simulink model "Simulation_NoVI"  (R2022b)
settings: Solver=VariableStepAuto  StartTime=0.0  StopTime=25  RelTol=1e-3
values from neighbouring files (symbols this model uses):
  A = [0 1 1 1 ; 1 0 1 1 ; 1 1 0 1 ; 1 1 1 0]    [Primary_test1.m]    (also in init.mat = [0 1 1 1 1 0 1 1 1 1 0 1 ... (16 elements, 4x4)])
  C_f = 0.000112315*9    (= 0.001010835)    [Main.m]    (also in PSO_2paras.m = swarm(i,2); PSO_filter_2paras.m = swarm(i,2)/10000; Primary_test1.m; Script_18June.m = 0.0112315)
  f_c = 50e3    (= 50000)    [Main.m]    (also in Primary_test1.m; Script_18June.m; Script_23June.m; Script_5thJune.m)
  k = -0.5    [Main.m]    (also in Primary_test1.m; Savedata.m = 0.2909; Script_18June.m = 0.5; Script_23June.m)
  K_h11 = 0    [Main.m]    (also in PSO_HC.m = swarm(i,4); Primary_test1.m; Script_18June.m; Script_23June.m)
  K_h13 = 0    [Main.m]    (also in Primary_test1.m; Script_18June.m; Script_23June.m; Script_5thJune.m)
  K_h5 = 0    [Main.m]    (also in PSO_HC.m = swarm(i,1); Primary_test1.m = 1; Script_18June.m; Script_23June.m)
  K_h7 = 0    [Main.m]    (also in PSO_HC.m = swarm(i,2); Primary_test1.m; Script_18June.m; Script_23June.m)
  K_h9 = 0    [Main.m]    (also in PSO_HC.m = swarm(i,3); Script_18June.m; Script_23June.m; Script_5thJune.m)
  ki_pr = 160    [Main.m]    (also in PSO.m = swarm(i,2); Primary_test1.m; Savedata.m = 422.4716; Script_18June.m = 150)
  kL = 1e-7    (= 1e-07)    [Main.m]    (also in Primary_test1.m; Script_18June.m; Script_23June.m; Script_5thJune.m)
  Kp_pr = 1.7    [Main.m]    (also in PSO.m = swarm(i,1); Primary_test1.m; Savedata.m = 0.9028; Script_18June.m = 1)
  L_f = 0.000659829*1.4    (= 0.0009237606)    [Main.m]    (also in PSO_2paras.m = swarm(i,1); PSO_filter_2paras.m = swarm(i,1); Primary_test1.m; Script_18June.m = 0.000295603392)
  L_in1 = 0.35e-3    (= 0.00035)    [Main.m]    (also in Primary_test1.m; Script_18June.m; Script_23June.m; Script_5thJune.m)
  L_in2 = 0.35e-3    (= 0.00035)    [Main.m]    (also in Primary_test1.m; Script_18June.m; Script_23June.m; Script_5thJune.m)
  L_in3 = 0.35e-3    (= 0.00035)    [Main.m]    (also in Primary_test1.m; Script_18June.m; Script_23June.m; Script_5thJune.m)
  L_in4 = 0.35e-3    (= 0.00035)    [Main.m]    (also in Primary_test1.m; Script_18June.m; Script_23June.m; Script_5thJune.m)
  lambda1 = 5.5*[1 1 0.8 0.8]'    [Primary_test1.m]    (also in init.mat = [5.5 5.5 4.4 4.4])
  lambda2 = 30.5*[0.8e-2 0.8e-2 0.5e-2 0.5e-2]'    [Primary_test1.m]    (also in init.mat = [0.244 0.244 0.1525 0.1525])
  lambda3 = 62.5*[1.5e-3 1.5e-3 1e-3 1.1e-3]'    [Primary_test1.m]    (also in init.mat = [0.09375 0.09375 0.0625 0.06875])
  LD_ref1 = 100e-6    (= 0.0001)    [Main.m]    (also in Primary_test1.m; Script_18June.m = 5e-05; Script_23June.m = 1e-05; Script_5thJune.m = 1e-05)
  lo_co = 0.1    [Main.m]    (also in Primary_test1.m; Script_18June.m; Script_23June.m; Script_5thJune.m)
  load_off = 10    [Main.m]    (also in Primary_test1.m = 2; Script_18June.m = 28; Script_23June.m = 28; Script_5thJune.m)
  load_on = 0.21    [Main.m]    (also in Primary_test1.m = 1; Script_18June.m; Script_23June.m; Script_5thJune.m)
  m_p1 = 9.4e-5/droopDivide    (= 9.4e-06)    [Main.m]    (also in Primary_test1.m; Script_18June.m = 9.4e-05; Script_23June.m = 9.4e-05; Script_5thJune.m = 5e-05)
  m_p2 = 9.4e-5/droopDivide    (= 9.4e-06)    [Main.m]    (also in Primary_test1.m; Script_18June.m = 9.4e-05; Script_23June.m = 9.4e-05; Script_5thJune.m = 5e-05)
  m_p3 = 11.4e-5/droopDivide    (= 1.14e-05)    [Main.m]    (also in Primary_test1.m; Script_18June.m = 0.000114; Script_23June.m = 0.000114; Script_5thJune.m = 6.42857142857e-05)
  m_p4 = 11.4e-5/droopDivide    (= 1.14e-05)    [Main.m]    (also in Primary_test1.m; Script_18June.m = 0.000114; Script_23June.m = 0.000114; Script_5thJune.m = 6.42857142857e-05)
  N = 2    [Primary_test1.m]    (also in init.mat)
  n_q1 = 1.3e-3/droopDivide2    (= 6.5e-05)    [Main.m]    (also in Primary_test1.m; Script_18June.m; Script_23June.m; Script_5thJune.m = 0.2)
  n_q2 = 1.3e-3/droopDivide2    (= 6.5e-05)    [Main.m]    (also in Primary_test1.m; Script_18June.m; Script_23June.m; Script_5thJune.m = 0.2)
  n_q3 = 1.5e-3/droopDivide2    (= 7.5e-05)    [Main.m]    (also in Primary_test1.m; Script_18June.m; Script_23June.m; Script_5thJune.m = 0.257142857143)
  n_q4 = 1.5e-3/droopDivide2    (= 7.5e-05)    [Main.m]    (also in Primary_test1.m; Script_18June.m; Script_23June.m; Script_5thJune.m = 0.257142857143)
  Pmax = [45e3 45e3 37e3 37e3]'    [Primary_test1.m]    (also in init.mat = [45000 45000 37000 37000])
  PMW = V_nom/0.55    [Main.m]    (also in Primary_test1.m; Script_18June.m = V_nom/0.4; Script_23June.m; Script_5thJune.m = 220*sqrt(2))
  R_f = 0.35    [Main.m]    (also in PSO_filter_2paras.m = 10*L_f; Primary_test1.m; Savedata.m = 0.249593207053; Script_18June.m = 0.1)
  R_in1 = 0.03    [Main.m]    (also in Primary_test1.m; Script_18June.m; Script_23June.m; Script_5thJune.m)
  R_in2 = 0.03    [Main.m]    (also in Primary_test1.m; Script_18June.m; Script_23June.m; Script_5thJune.m)
  R_in3 = 0.03    [Main.m]    (also in Primary_test1.m; Script_18June.m; Script_23June.m; Script_5thJune.m)
  R_in4 = 0.03    [Main.m]    (also in Primary_test1.m; Script_18June.m; Script_23June.m; Script_5thJune.m)
  time_thresh = 0.2    [Main.m]    (also in Primary_test1.m; Script_18June.m; Script_23June.m; Script_5thJune.m)
  Ts = 10e-6    (= 1e-05)    [Main.m]    (also in Primary_test1.m; Script_18June.m; Script_23June.m; Script_5thJune.m)
  Tsamp = 0.1    [Primary_test1.m]    (also in init.mat)
  V_nom = 220*sqrt(2)    [Main.m]    (also in Primary_test1.m; Script_18June.m; Script_23June.m; Script_5thJune.m)
  Vdc = 600    [Main.m]    (also in Primary_test1.m; Script_18June.m; Script_23June.m; Script_5thJune.m)
  w_c_high = 2*pi*50    (= 314.159265359)    [Main.m]    (also in Primary_test1.m; Script_18June.m = 307.876080052; Script_23June.m; Script_5thJune.m = 307.876080052)
  w_nom = 2*pi*f    (= 314.159265359)    [Main.m]    (also in Primary_test1.m; Script_18June.m; Script_23June.m; Script_5thJune.m)
  wc_hc = 1    [Main.m]    (also in Primary_test1.m; Script_18June.m = 0.3; Script_23June.m; Script_5thJune.m = 0.3)
  wc_pr = 3    [Main.m]    (also in PSO.m = swarm(i,3); Primary_test1.m; Savedata.m = 1.36672; Script_18June.m = 1.5)
undefined symbols (not defined in the file or in its folder): DiscIntNeverNeededParam, i
libraries: eeGeneralControl x16, spsThreePhaseSeriesRLCBranchLib x15, spsThreePhaseVIMeasurementLib x12, spsabctoAlphaBetaZeroLib x12, spsabctodq0Lib x12, slpidlib x8, spsThreePhaseSeriesRLCLoadLib x6, spsThreePhaseBreakerLib x6, spsDCVoltageSourceLib x4, spsAlphaBetaZerotoabcLib x4, spsSeriesRLCBranchLib x4, spsTriangleGeneratorLib x4
(part 2 of 5)

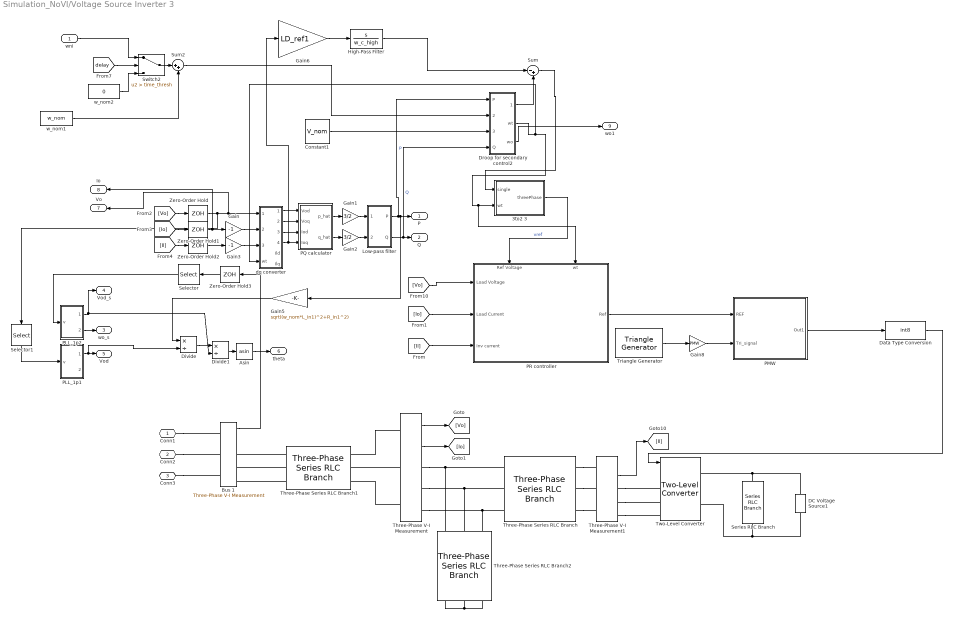
== system Simulation_NoVI/Voltage Source Inverter 3 ==
  wni : Inport
  3to2 3 : Subsystem
  Asin : Trigonometry  Operator=asin
  Bus 1 : spsThreePhaseVIMeasurementLib/Three-Phase V-I Measurement  VoltageMeasurement=phase-to-ground  SetLabelV=off  LabelV=Vbus  Vpu=off  VpuLL=off  CurrentMeasurement=yes  SetLabelI=off  LabelI=Ibus  Ipu=off  Pbase=100e6  Vbase=380  OutputType=Complex  PhasorSimulation=off  PSBequivalent=0
  Constant1 : Constant  Value=V_nom
  DC Voltage Source1 : spsDCVoltageSourceLib/DC Voltage Source  Amplitude=Vdc  Measurements=None
  Data Type Conversion : DataTypeConversion  OutDataTypeStr=int8  SaturateOnIntegerOverflow=off  RndMeth=Floor
  Divide : Product  Inputs=*/
  Divide1 : Product  Inputs=*/
  Droop for secondary control2 : Subsystem
  Gain : Gain  Gain=-1
  Gain1 : Gain  Gain=3/2
  Gain2 : Gain  Gain=3/2
  Gain3 : Gain  Gain=-1
  Gain5 : Gain  Gain=sqrt((w_nom*L_in1)^2+R_in1^2)
  Gain6 : Gain  Gain=LD_ref1
  Gain8 : Gain  Gain=PMW
  High-Pass Filter : TransferFcn  Numerator=[1 0]  Denominator=w_c_high
  Low-pass filter : Subsystem
  PLL_1p1 : Subsystem  SystemSampleTime=10*Ts
      settings: MinAlgLoopOccurrences=on
  PLL_1p2 : Subsystem  SystemSampleTime=10*Ts
      settings: MinAlgLoopOccurrences=on
  PMW : Subsystem
  PQ calculator : Subsystem
  PR controller : Subsystem
      settings: PortSchema="{\"entries\":[{\"content\":{\"sides\":[{\"content\":{\"connectorIds\":[\"In1\",\"In2\",\"In3\"]},\"type\":\"ConnectorPlacement.EquallySpacedRectSide\",\"uuid\":\"7320bc60-546b-444c-8acd-b3f08639d81a\"},{\"content\":{\"connectorIds\":[\"Out1\"],\"side\":\"RIGHT\"},\"type\":\"ConnectorPlacement.EquallySpacedRectSide\",\"uuid\":\"69cfd51f-d98e-4566-bb44-68be2b580a1e\"},{\"content\":{\"connectorIds\":[\"In4\",\"In5\"],\"side\":\"TOP\"},\"type\":\"ConnectorPlacement.EquallySpacedRectSide\",\"uuid\":\"122ed5ae-7585-404b-87e2-f9556d95c9dc\"}]},\"type\":\"ConnectorPlacement.EquallySpacedConnector\",\"uuid\":\"74384932-3814-4f3d-adae-cd0ccfea3412\"}],\"packageUris\":[\"http://schema.mathworks.com/mf0/Connector/R2020b\"],\"version\":\"1.0\"}"
  Selector : Selector  InputPortWidth=3  IndexOptions=Index vector (dialog)  Indices=[1]  OutputSizes=1
  Selector1 : Selector  InputPortWidth=3  IndexOptions=Index vector (dialog)  Indices=[1]  OutputSizes=1
  Series RLC Branch : spsSeriesRLCBranchLib/Series RLC Branch  LConnTagsString=__new0  RConnTagsString=__new0  BranchType=RC  Resistance=30  Inductance=1e-3  SetiL0=off  InitialCurrent=0  Capacitance=80e-6  Setx0=off  InitialVoltage=0  Measurements=None
  Sum : Sum  Inputs=|-+
  Sum2 : Sum  Inputs=|++
  Switch2 : Switch  Criteria=u2 > Threshold  Threshold=time_thresh  SaturateOnIntegerOverflow=off  InputSameDT=off
  Three-Phase Series RLC Branch : spsThreePhaseSeriesRLCBranchLib/Three-Phase Series RLC Branch  LConnTagsString=A|B|C  RConnTagsString=A|B|C  BranchType=RL  Resistance=R_f  Inductance=L_f  Capacitance=1e-6  Measurements=None
  Three-Phase Series RLC Branch1 : spsThreePhaseSeriesRLCBranchLib/Three-Phase Series RLC Branch  LConnTagsString=A|B|C  RConnTagsString=A|B|C  BranchType=RL  Resistance=R_in  Inductance=L_in  Capacitance=1e-6  Measurements=None
  Three-Phase Series RLC Branch2 : spsThreePhaseSeriesRLCBranchLib/Three-Phase Series RLC Branch  LConnTagsString=A|B|C  RConnTagsString=A|B|C  BranchType=C  Resistance=R_f  Inductance=1e-3  Capacitance=C_f  Measurements=None
  Three-Phase V-I Measurement : spsThreePhaseVIMeasurementLib/Three-Phase V-I Measurement  VoltageMeasurement=phase-to-ground  SetLabelV=off  LabelV=Vo1  Vpu=off  VpuLL=off  CurrentMeasurement=yes  SetLabelI=off  LabelI=Io1  Ipu=off  Pbase=100e6  Vbase=500e3  OutputType=Complex  PhasorSimulation=off  PSBequivalent=0
  Three-Phase V-I Measurement1 : spsThreePhaseVIMeasurementLib/Three-Phase V-I Measurement  VoltageMeasurement=phase-to-ground  SetLabelV=off  LabelV=Vl2  Vpu=off  VpuLL=off  CurrentMeasurement=yes  SetLabelI=off  LabelI=Il2  Ipu=off  Pbase=100e6  Vbase=500e3  OutputType=Complex  PhasorSimulation=off  PSBequivalent=0
  Triangle Generator : spsTriangleGeneratorLib/Triangle Generator  Freq=5000  Phase=90  Ts=0
  Two-Level Converter : spsTwoLevelConverterLib/Two-Level Converter  ModelType=Switching devices  Ron=1e-3  Rs=1e6  Cs=inf  Vforward=[0,0]  Ron_Diode=1e-3  Rs_Diode=1e6  Cs_Diode=inf  Vf_Diode=1e-3  Rs_CurrentSource=inf  Ron_ACsource=1e-3
  Zero-Order Hold : ZeroOrderHold  SampleTime=modT
  Zero-Order Hold1 : ZeroOrderHold  SampleTime=modT
  Zero-Order Hold2 : ZeroOrderHold  SampleTime=modT
  Zero-Order Hold3 : ZeroOrderHold  SampleTime=-1
  dq converter : Subsystem
  w_nom1 : Constant  Value=w_nom
  w_nom2 : Constant  Value=0
  Conn1 : PMIOPort  Side=Left
  Conn2 : PMIOPort  Port=2  Side=Left
  Conn3 : PMIOPort  Port=3  Side=Left
  P : Outport
  Q : Outport  Port=2
  wo_s : Outport  Port=3
  Vod_s : Outport  Port=4
  Vod : Outport  Port=5
  theta : Outport  Port=6
  Vo : Outport  Port=7
  Io : Outport  Port=8
  wo1 : Outport  Port=9
  wires:
  Three-Phase V-I Measurement/1 -> [Vo]
  Three-Phase V-I Measurement/2 -> [Io]
  Three-Phase V-I Measurement1/2 -> [Il]
  [Il] -> Zero-Order Hold2/1
  Gain1/1 -> Low-pass filter/1(p_hat)
  PQ calculator/2(q_hat) -> Gain2/1
  Gain2/1 -> Low-pass filter/2(q_hat)
  dq converter/1(Vod) -> PQ calculator/1(Vod)
  Low-pass filter/2(Q) -> Droop for secondary control2/4(Q), Q/1  "Q"
  Gain3/1 -> dq converter/3(Ildq)
  Low-pass filter/1(P) -> Droop for secondary control2/1(P), Gain5/1, P/1  "P"
  Gain/1 -> dq converter/2(Iodq)
  [Io] -> Zero-Order Hold1/1
  Zero-Order Hold2/1 -> Gain3/1
  [Vo] -> Zero-Order Hold/1
  dq converter/3(Iod) -> PQ calculator/3(Iod)
  Zero-Order Hold1/1 -> Gain/1, Io/1
  dq converter/2(Voq) -> PQ calculator/2(Voq)
  PQ calculator/1(p_hat) -> Gain1/1
  [Il] -> PR controller/3(Inv current)
  Bus 1/1 -> Zero-Order Hold3/1
  PMW/1(Out1) -> Data Type Conversion/1
  Data Type Conversion/1 -> Two-Level Converter/1
  dq converter/4(Ioq) -> Gain6/1, PQ calculator/4(Ioq)
  Gain6/1 -> High-Pass Filter/1
  Droop for secondary control2/2(wt) -> PR controller/5(wt), 3to2 3/2("wt "), dq converter/4(wt)
  Droop for secondary control2/3(wo) -> wo1/1
  [Vo] -> PR controller/1(Load Voltage)
  Constant1/1 -> Droop for secondary control2/3(V_nom)
  Sum/1 -> 3to2 3/1("single ")
  3to2 3/1(threePhase) -> PR controller/4(Ref Voltage)  "vref"
  Zero-Order Hold3/1 -> Selector/1
  Selector1/1 -> PLL_1p1/1(v)
  Selector/1 -> PLL_1p2/1(v)
  PLL_1p2/2(omega) -> wo_s/1
  Gain5/1 -> Divide/1
  Divide/1 -> Divide1/1
  PLL_1p2/1(v_dq) -> Divide1/2, Vod_s/1
  PLL_1p1/1(v_dq) -> Divide/2, Vod/1
  Divide1/1 -> Asin/1
  Asin/1 -> theta/1
  Zero-Order Hold/1 -> Selector1/1, Vo/1, dq converter/1(Vodq)
  Triangle Generator/1 -> Gain8/1
  Gain8/1 -> PMW/2(Tri_signal)
  Droop for secondary control2/1(Vref) -> Sum/2
  High-Pass Filter/1 -> Sum/1
  PR controller/1(Ref) -> PMW/1(REF)
  Sum2/1 -> Droop for secondary control2/2(w_nom)
  w_nom2/1 -> Switch2/3
  wni/1 -> Switch2/1
  [delay] -> Switch2/2
  w_nom1/1 -> Sum2/2
  Switch2/1 -> Sum2/1
  [Io] -> PR controller/2(Load Current)
  connections:
  Conn3/RConn1 -- Bus 1/LConn3
  Conn1/RConn1 -- Bus 1/LConn1
  Conn2/RConn1 -- Bus 1/LConn2
  Two-Level Converter/RConn1 -- DC Voltage Source1/RConn1 -- Series RLC Branch/LConn1
  DC Voltage Source1/LConn1 -- Two-Level Converter/RConn2 -- Series RLC Branch/RConn1
  Three-Phase V-I Measurement1/RConn1 -- Two-Level Converter/LConn1
  Three-Phase V-I Measurement1/RConn2 -- Two-Level Converter/LConn2
  Three-Phase V-I Measurement1/RConn3 -- Two-Level Converter/LConn3
  Three-Phase Series RLC Branch/RConn2 -- Three-Phase V-I Measurement1/LConn2
  Three-Phase Series RLC Branch/RConn1 -- Three-Phase V-I Measurement1/LConn1
  Three-Phase Series RLC Branch/RConn3 -- Three-Phase V-I Measurement1/LConn3
  Three-Phase Series RLC Branch2/RConn1 -- Three-Phase Series RLC Branch2/RConn3 -- Three-Phase Series RLC Branch2/RConn2
  Three-Phase V-I Measurement/RConn2 -- Three-Phase Series RLC Branch2/LConn2 -- Three-Phase Series RLC Branch/LConn2
  Three-Phase V-I Measurement/RConn1 -- Three-Phase Series RLC Branch/LConn1 -- Three-Phase Series RLC Branch2/LConn1
  Three-Phase V-I Measurement/RConn3 -- Three-Phase Series RLC Branch2/LConn3 -- Three-Phase Series RLC Branch/LConn3
  Three-Phase V-I Measurement/LConn1 -- Three-Phase Series RLC Branch1/RConn1
  Three-Phase V-I Measurement/LConn2 -- Three-Phase Series RLC Branch1/RConn2
  Three-Phase V-I Measurement/LConn3 -- Three-Phase Series RLC Branch1/RConn3
  Three-Phase Series RLC Branch1/LConn1 -- Bus 1/RConn1
  Three-Phase Series RLC Branch1/LConn2 -- Bus 1/RConn2
  Three-Phase Series RLC Branch1/LConn3 -- Bus 1/RConn3

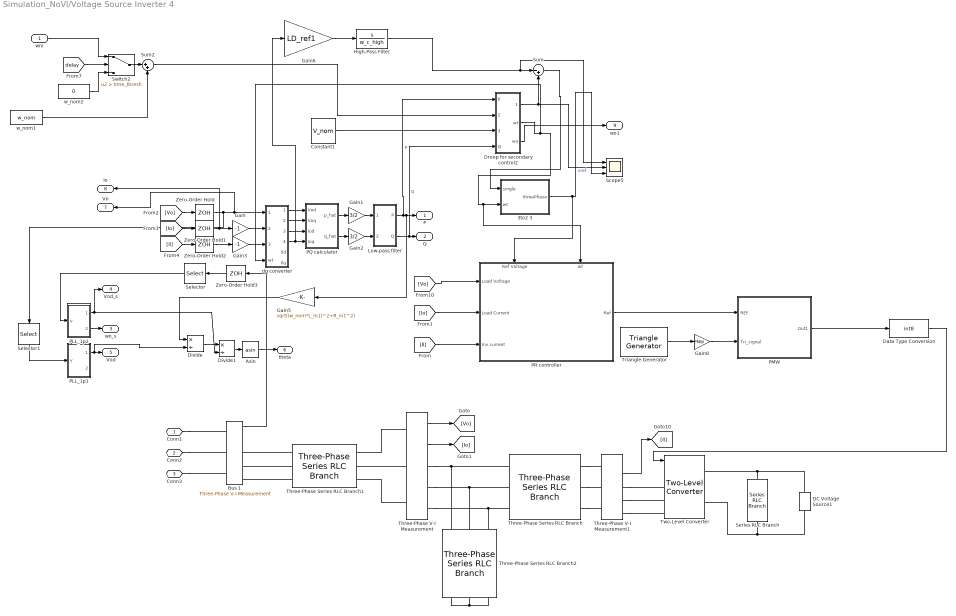
== system Simulation_NoVI/Voltage Source Inverter 4 ==
  wni : Inport
  3to2 3 : Subsystem
  Asin : Trigonometry  Operator=asin
  Bus 1 : spsThreePhaseVIMeasurementLib/Three-Phase V-I Measurement  VoltageMeasurement=phase-to-ground  SetLabelV=off  LabelV=Vbus  Vpu=off  VpuLL=off  CurrentMeasurement=yes  SetLabelI=off  LabelI=Ibus  Ipu=off  Pbase=100e6  Vbase=380  OutputType=Complex  PhasorSimulation=off  PSBequivalent=0
  Constant1 : Constant  Value=V_nom
  DC Voltage Source1 : spsDCVoltageSourceLib/DC Voltage Source  Amplitude=Vdc  Measurements=None
  Data Type Conversion : DataTypeConversion  OutDataTypeStr=int8  SaturateOnIntegerOverflow=off  RndMeth=Floor
  Divide : Product  Inputs=*/
  Divide1 : Product  Inputs=*/
  Droop for secondary control2 : Subsystem
  Gain : Gain  Gain=-1
  Gain1 : Gain  Gain=3/2
  Gain2 : Gain  Gain=3/2
  Gain3 : Gain  Gain=-1
  Gain5 : Gain  Gain=sqrt((w_nom*L_in1)^2+R_in1^2)
  Gain6 : Gain  Gain=LD_ref1
  Gain8 : Gain  Gain=PMW
  High-Pass Filter : TransferFcn  Numerator=[1 0]  Denominator=w_c_high
  Low-pass filter : Subsystem
  PLL_1p1 : Subsystem  SystemSampleTime=10*Ts
      settings: MinAlgLoopOccurrences=on
  PLL_1p2 : Subsystem  SystemSampleTime=10*Ts
      settings: MinAlgLoopOccurrences=on
  PMW : Subsystem
  PQ calculator : Subsystem
  PR controller : Subsystem
      settings: PortSchema="{\"entries\":[{\"content\":{\"sides\":[{\"content\":{\"connectorIds\":[\"In1\",\"In2\",\"In3\"]},\"type\":\"ConnectorPlacement.EquallySpacedRectSide\",\"uuid\":\"7320bc60-546b-444c-8acd-b3f08639d81a\"},{\"content\":{\"connectorIds\":[\"Out1\"],\"side\":\"RIGHT\"},\"type\":\"ConnectorPlacement.EquallySpacedRectSide\",\"uuid\":\"69cfd51f-d98e-4566-bb44-68be2b580a1e\"},{\"content\":{\"connectorIds\":[\"In4\",\"In5\"],\"side\":\"TOP\"},\"type\":\"ConnectorPlacement.EquallySpacedRectSide\",\"uuid\":\"122ed5ae-7585-404b-87e2-f9556d95c9dc\"}]},\"type\":\"ConnectorPlacement.EquallySpacedConnector\",\"uuid\":\"74384932-3814-4f3d-adae-cd0ccfea3412\"}],\"packageUris\":[\"http://schema.mathworks.com/mf0/Connector/R2020b\"],\"version\":\"1.0\"}"
  Scope5 : Scope  NumInputPorts=3
  Selector : Selector  InputPortWidth=3  IndexOptions=Index vector (dialog)  Indices=[1]  OutputSizes=1
  Selector1 : Selector  InputPortWidth=3  IndexOptions=Index vector (dialog)  Indices=[1]  OutputSizes=1
  Series RLC Branch : spsSeriesRLCBranchLib/Series RLC Branch  LConnTagsString=__new0  RConnTagsString=__new0  BranchType=RC  Resistance=30  Inductance=1e-3  SetiL0=off  InitialCurrent=0  Capacitance=80e-6  Setx0=off  InitialVoltage=0  Measurements=None
  Sum : Sum  Inputs=|-+
  Sum2 : Sum  Inputs=|++
  Switch2 : Switch  Criteria=u2 > Threshold  Threshold=time_thresh  SaturateOnIntegerOverflow=off  InputSameDT=off
  Three-Phase Series RLC Branch : spsThreePhaseSeriesRLCBranchLib/Three-Phase Series RLC Branch  LConnTagsString=A|B|C  RConnTagsString=A|B|C  BranchType=RL  Resistance=R_f  Inductance=L_f  Capacitance=1e-6  Measurements=None
  Three-Phase Series RLC Branch1 : spsThreePhaseSeriesRLCBranchLib/Three-Phase Series RLC Branch  LConnTagsString=A|B|C  RConnTagsString=A|B|C  BranchType=RL  Resistance=R_in  Inductance=L_in  Capacitance=1e-6  Measurements=None
  Three-Phase Series RLC Branch2 : spsThreePhaseSeriesRLCBranchLib/Three-Phase Series RLC Branch  LConnTagsString=A|B|C  RConnTagsString=A|B|C  BranchType=C  Resistance=R_f  Inductance=1e-3  Capacitance=C_f  Measurements=None
  Three-Phase V-I Measurement : spsThreePhaseVIMeasurementLib/Three-Phase V-I Measurement  VoltageMeasurement=phase-to-ground  SetLabelV=off  LabelV=Vo1  Vpu=off  VpuLL=off  CurrentMeasurement=yes  SetLabelI=off  LabelI=Io1  Ipu=off  Pbase=100e6  Vbase=500e3  OutputType=Complex  PhasorSimulation=off  PSBequivalent=0
  Three-Phase V-I Measurement1 : spsThreePhaseVIMeasurementLib/Three-Phase V-I Measurement  VoltageMeasurement=phase-to-ground  SetLabelV=off  LabelV=Vl2  Vpu=off  VpuLL=off  CurrentMeasurement=yes  SetLabelI=off  LabelI=Il2  Ipu=off  Pbase=100e6  Vbase=500e3  OutputType=Complex  PhasorSimulation=off  PSBequivalent=0
  Triangle Generator : spsTriangleGeneratorLib/Triangle Generator  Freq=5000  Phase=90  Ts=0
  Two-Level Converter : spsTwoLevelConverterLib/Two-Level Converter  ModelType=Switching devices  Ron=1e-3  Rs=1e6  Cs=inf  Vforward=[0,0]  Ron_Diode=1e-3  Rs_Diode=1e6  Cs_Diode=inf  Vf_Diode=1e-3  Rs_CurrentSource=inf  Ron_ACsource=1e-3
  Zero-Order Hold : ZeroOrderHold  SampleTime=modT
  Zero-Order Hold1 : ZeroOrderHold  SampleTime=modT
  Zero-Order Hold2 : ZeroOrderHold  SampleTime=modT
  Zero-Order Hold3 : ZeroOrderHold  SampleTime=-1
  dq converter : Subsystem
  w_nom1 : Constant  Value=w_nom
  w_nom2 : Constant  Value=0
  Conn1 : PMIOPort  Side=Left
  Conn2 : PMIOPort  Port=2  Side=Left
  Conn3 : PMIOPort  Port=3  Side=Left
  P : Outport
  Q : Outport  Port=2
  wo_s : Outport  Port=3
  Vod_s : Outport  Port=4
  Vod : Outport  Port=5
  theta : Outport  Port=6
  Vo : Outport  Port=7
  Io : Outport  Port=8
  wo1 : Outport  Port=9
  wires:
  Three-Phase V-I Measurement/1 -> [Vo]
  Three-Phase V-I Measurement/2 -> [Io]
  Three-Phase V-I Measurement1/2 -> [Il]
  [Il] -> Zero-Order Hold2/1
  Gain1/1 -> Low-pass filter/1(p_hat)
  PQ calculator/2(q_hat) -> Gain2/1
  Gain2/1 -> Low-pass filter/2(q_hat)
  dq converter/1(Vod) -> PQ calculator/1(Vod)
  Low-pass filter/2(Q) -> Droop for secondary control2/4(Q), Q/1  "Q"
  Gain3/1 -> dq converter/3(Ildq)
  Low-pass filter/1(P) -> Droop for secondary control2/1(P), Gain5/1, P/1  "P"
  Gain/1 -> dq converter/2(Iodq)
  [Io] -> Zero-Order Hold1/1
  Zero-Order Hold2/1 -> Gain3/1
  [Vo] -> Zero-Order Hold/1
  dq converter/3(Iod) -> PQ calculator/3(Iod)
  Zero-Order Hold1/1 -> Gain/1, Io/1
  dq converter/2(Voq) -> PQ calculator/2(Voq)
  PQ calculator/1(p_hat) -> Gain1/1
  [Il] -> PR controller/3(Inv current)
  Bus 1/1 -> Zero-Order Hold3/1
  PMW/1(Out1) -> Data Type Conversion/1
  Data Type Conversion/1 -> Two-Level Converter/1
  [Io] -> PR controller/2(Load Current)
  dq converter/4(Ioq) -> Gain6/1, PQ calculator/4(Ioq)
  Gain6/1 -> High-Pass Filter/1
  Droop for secondary control2/2(wt) -> PR controller/5(wt), 3to2 3/2("wt "), dq converter/4(wt)
  Droop for secondary control2/3(wo) -> wo1/1
  [Vo] -> PR controller/1(Load Voltage)
  Constant1/1 -> Droop for secondary control2/3(V_nom)
  Sum/1 -> 3to2 3/1("single ")
  3to2 3/1(threePhase) -> PR controller/4(Ref Voltage), Scope5/3  "vref"
  Zero-Order Hold3/1 -> Selector/1
  Selector1/1 -> PLL_1p1/1(v)
  Selector/1 -> PLL_1p2/1(v)
  PLL_1p2/2(omega) -> wo_s/1
  Gain5/1 -> Divide/1
  Divide/1 -> Divide1/1
  PLL_1p2/1(v_dq) -> Divide1/2, Vod_s/1
  PLL_1p1/1(v_dq) -> Divide/2, Vod/1
  Divide1/1 -> Asin/1
  Asin/1 -> theta/1
  Zero-Order Hold/1 -> Selector1/1, Vo/1, dq converter/1(Vodq)
  Triangle Generator/1 -> Gain8/1
  Gain8/1 -> PMW/2(Tri_signal)
  Droop for secondary control2/1(Vref) -> Scope5/2, Sum/2
  High-Pass Filter/1 -> Sum/1, Scope5/1
  PR controller/1(Ref) -> PMW/1(REF)
  Sum2/1 -> Droop for secondary control2/2(w_nom)
  w_nom2/1 -> Switch2/3
  wni/1 -> Switch2/1
  [delay] -> Switch2/2
  w_nom1/1 -> Sum2/2
  Switch2/1 -> Sum2/1
  connections:
  Conn3/RConn1 -- Bus 1/LConn3
  Conn1/RConn1 -- Bus 1/LConn1
  Conn2/RConn1 -- Bus 1/LConn2
  Two-Level Converter/RConn1 -- DC Voltage Source1/RConn1 -- Series RLC Branch/LConn1
  DC Voltage Source1/LConn1 -- Two-Level Converter/RConn2 -- Series RLC Branch/RConn1
  Three-Phase V-I Measurement1/RConn1 -- Two-Level Converter/LConn1
  Three-Phase V-I Measurement1/RConn2 -- Two-Level Converter/LConn2
  Three-Phase V-I Measurement1/RConn3 -- Two-Level Converter/LConn3
  Three-Phase Series RLC Branch/RConn2 -- Three-Phase V-I Measurement1/LConn2
  Three-Phase Series RLC Branch/RConn1 -- Three-Phase V-I Measurement1/LConn1
  Three-Phase Series RLC Branch/RConn3 -- Three-Phase V-I Measurement1/LConn3
  Three-Phase Series RLC Branch2/RConn1 -- Three-Phase Series RLC Branch2/RConn3 -- Three-Phase Series RLC Branch2/RConn2
  Three-Phase V-I Measurement/RConn2 -- Three-Phase Series RLC Branch2/LConn2 -- Three-Phase Series RLC Branch/LConn2
  Three-Phase V-I Measurement/RConn1 -- Three-Phase Series RLC Branch/LConn1 -- Three-Phase Series RLC Branch2/LConn1
  Three-Phase V-I Measurement/RConn3 -- Three-Phase Series RLC Branch2/LConn3 -- Three-Phase Series RLC Branch/LConn3
  Three-Phase V-I Measurement/LConn1 -- Three-Phase Series RLC Branch1/RConn1
  Three-Phase V-I Measurement/LConn2 -- Three-Phase Series RLC Branch1/RConn2
  Three-Phase V-I Measurement/LConn3 -- Three-Phase Series RLC Branch1/RConn3
  Three-Phase Series RLC Branch1/LConn1 -- Bus 1/RConn1
  Three-Phase Series RLC Branch1/LConn2 -- Bus 1/RConn2
  Three-Phase Series RLC Branch1/LConn3 -- Bus 1/RConn3

== system Simulation_NoVI/MPC-based Secondary Controller/Subsystem ==
  In1 : Inport
  In2 : Inport  Port=2
  In3 : Inport  Port=3
  In4 : Inport  Port=4
  In5 : Inport  Port=5
  In6 : Inport  Port=6
  Demux : Demux  Outputs=6
  Mux : Mux  Inputs=6
  Rate Transition : RateTransition  InitialCondition=10e-6  OutPortSampleTime=Tsamp
  Out1 : Outport
  Out2 : Outport  Port=2
  Out3 : Outport  Port=3
  Out4 : Outport  Port=4
  Out5 : Outport  Port=5
  Out6 : Outport  Port=6
  wires:
  In6/1 -> Mux/6
  Mux/1 -> Rate Transition/1
  Demux/5 -> Out5/1
  Rate Transition/1 -> Demux/1
  In5/1 -> Mux/5
  Demux/3 -> Out3/1
  In3/1 -> Mux/3
  Demux/4 -> Out4/1
  In4/1 -> Mux/4
  Demux/2 -> Out2/1
  Demux/1 -> Out1/1
  Demux/6 -> Out6/1
  In2/1 -> Mux/2
  In1/1 -> Mux/1

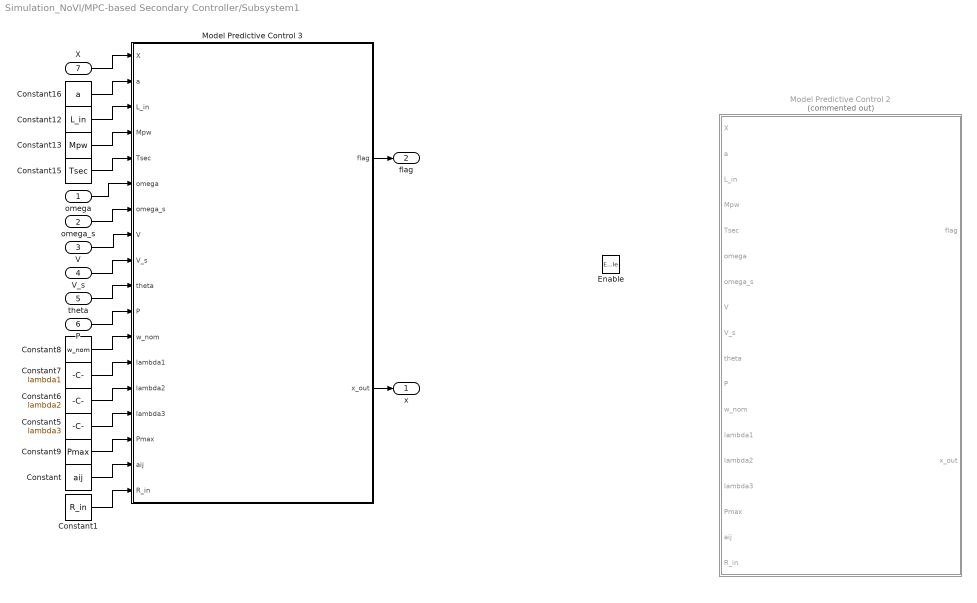
== system Simulation_NoVI/MPC-based Secondary Controller/Subsystem1 ==
  omega : Inport
  omega_s : Inport  Port=2
  V : Inport  Port=3
  V_s : Inport  Port=4
  theta : Inport  Port=5
  P : Inport  Port=6
  X : Inport  Port=7
  Enable : EnablePort
  Constant : Constant  Value=aij
  Constant1 : Constant  Value=R_in
  Constant12 : Constant  Value=L_in
  Constant13 : Constant  Value=Mpw
  Constant15 : Constant  Value=Tsec
  Constant16 : Constant  Value=a
  Constant5 : Constant  Value=lambda3
  Constant6 : Constant  Value=lambda2
  Constant7 : Constant  Value=lambda1
  Constant8 : Constant  Value=w_nom
  Constant9 : Constant  Value=Pmax
  Model Predictive Control 2 : MATLAB Function  Commented=on  SystemSampleTime=Tsamp
      settings: MinAlgLoopOccurrences=on
  Model Predictive Control 3 : MATLAB Function  SystemSampleTime=Tsamp
      settings: MinAlgLoopOccurrences=on
  x : Outport
  flag : Outport  Port=2
  wires:
  Constant8/1 -> Model Predictive Control 3/12(w_nom)
  V_s/1 -> Model Predictive Control 3/9(V_s)
  P/1 -> Model Predictive Control 3/11(P)
  omega_s/1 -> Model Predictive Control 3/7(omega_s)
  Constant/1 -> Model Predictive Control 3/17(aij)
  Constant15/1 -> Model Predictive Control 3/5(Tsec)
  omega/1 -> Model Predictive Control 3/6(omega)
  Model Predictive Control 3/2(x_out) -> x/1
  Constant16/1 -> Model Predictive Control 3/2(a)
  Constant13/1 -> Model Predictive Control 3/4(Mpw)
  X/1 -> Model Predictive Control 3/1(X)
  Constant12/1 -> Model Predictive Control 3/3(L_in)
  Constant9/1 -> Model Predictive Control 3/16(Pmax)
  Constant7/1 -> Model Predictive Control 3/13(lambda1)
  Constant5/1 -> Model Predictive Control 3/15(lambda3)
  V/1 -> Model Predictive Control 3/8(V)
  theta/1 -> Model Predictive Control 3/10(theta)
  Constant6/1 -> Model Predictive Control 3/14(lambda2)
  Model Predictive Control 3/1(flag) -> flag/1
  Constant1/1 -> Model Predictive Control 3/18(R_in)

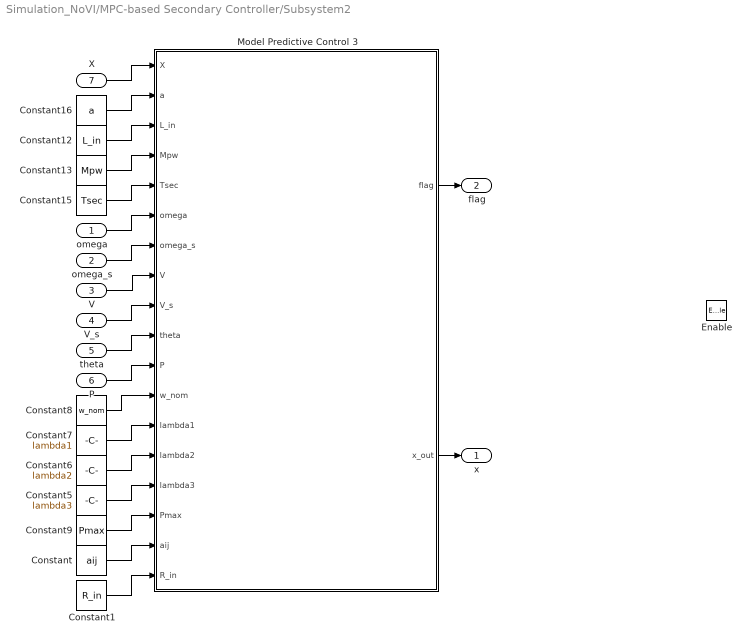
== system Simulation_NoVI/MPC-based Secondary Controller/Subsystem2 ==
  omega : Inport
  omega_s : Inport  Port=2
  V : Inport  Port=3
  V_s : Inport  Port=4
  theta : Inport  Port=5
  P : Inport  Port=6
  X : Inport  Port=7
  Enable : EnablePort
  Constant : Constant  Value=aij
  Constant1 : Constant  Value=R_in
  Constant12 : Constant  Value=L_in
  Constant13 : Constant  Value=Mpw
  Constant15 : Constant  Value=Tsec
  Constant16 : Constant  Value=a
  Constant5 : Constant  Value=lambda3
  Constant6 : Constant  Value=lambda2
  Constant7 : Constant  Value=lambda1
  Constant8 : Constant  Value=w_nom
  Constant9 : Constant  Value=Pmax
  Model Predictive Control 3 : MATLAB Function  SystemSampleTime=Tsamp
      settings: MinAlgLoopOccurrences=on
  x : Outport
  flag : Outport  Port=2
  wires:
  Constant8/1 -> Model Predictive Control 3/12(w_nom)
  V_s/1 -> Model Predictive Control 3/9(V_s)
  P/1 -> Model Predictive Control 3/11(P)
  omega_s/1 -> Model Predictive Control 3/7(omega_s)
  Constant/1 -> Model Predictive Control 3/17(aij)
  Constant15/1 -> Model Predictive Control 3/5(Tsec)
  omega/1 -> Model Predictive Control 3/6(omega)
  Model Predictive Control 3/2(x_out) -> x/1
  Constant16/1 -> Model Predictive Control 3/2(a)
  Constant13/1 -> Model Predictive Control 3/4(Mpw)
  X/1 -> Model Predictive Control 3/1(X)
  Constant12/1 -> Model Predictive Control 3/3(L_in)
  Constant9/1 -> Model Predictive Control 3/16(Pmax)
  Constant7/1 -> Model Predictive Control 3/13(lambda1)
  Constant5/1 -> Model Predictive Control 3/15(lambda3)
  V/1 -> Model Predictive Control 3/8(V)
  theta/1 -> Model Predictive Control 3/10(theta)
  Constant6/1 -> Model Predictive Control 3/14(lambda2)
  Model Predictive Control 3/1(flag) -> flag/1
  Constant1/1 -> Model Predictive Control 3/18(R_in)

== system Simulation_NoVI/MPC-based Secondary Controller/Subsystem3 ==
  omega : Inport
  omega_s : Inport  Port=2
  V : Inport  Port=3
  V_s : Inport  Port=4
  theta : Inport  Port=5
  P : Inport  Port=6
  X : Inport  Port=7
  Enable : EnablePort
  Constant : Constant  Value=aij
  Constant1 : Constant  Value=R_in
  Constant12 : Constant  Value=L_in
  Constant13 : Constant  Value=Mpw
  Constant15 : Constant  Value=Tsec
  Constant16 : Constant  Value=a
  Constant5 : Constant  Value=lambda3
  Constant6 : Constant  Value=lambda2
  Constant7 : Constant  Value=lambda1
  Constant8 : Constant  Value=w_nom
  Constant9 : Constant  Value=Pmax
  Model Predictive Control 3 : MATLAB Function  SystemSampleTime=Tsamp
      settings: MinAlgLoopOccurrences=on
  x : Outport
  flag : Outport  Port=2
  wires:
  Constant8/1 -> Model Predictive Control 3/12(w_nom)
  V_s/1 -> Model Predictive Control 3/9(V_s)
  P/1 -> Model Predictive Control 3/11(P)
  omega_s/1 -> Model Predictive Control 3/7(omega_s)
  Constant/1 -> Model Predictive Control 3/17(aij)
  Constant15/1 -> Model Predictive Control 3/5(Tsec)
  omega/1 -> Model Predictive Control 3/6(omega)
  Model Predictive Control 3/2(x_out) -> x/1
  Constant16/1 -> Model Predictive Control 3/2(a)
  Constant13/1 -> Model Predictive Control 3/4(Mpw)
  X/1 -> Model Predictive Control 3/1(X)
  Constant12/1 -> Model Predictive Control 3/3(L_in)
  Constant9/1 -> Model Predictive Control 3/16(Pmax)
  Constant7/1 -> Model Predictive Control 3/13(lambda1)
  Constant5/1 -> Model Predictive Control 3/15(lambda3)
  V/1 -> Model Predictive Control 3/8(V)
  theta/1 -> Model Predictive Control 3/10(theta)
  Constant6/1 -> Model Predictive Control 3/14(lambda2)
  Model Predictive Control 3/1(flag) -> flag/1
  Constant1/1 -> Model Predictive Control 3/18(R_in)

== system Simulation_NoVI/MPC-based Secondary Controller/Subsystem4 ==
  omega : Inport
  omega_s : Inport  Port=2
  V : Inport  Port=3
  V_s : Inport  Port=4
  theta : Inport  Port=5
  P : Inport  Port=6
  X : Inport  Port=7
  Enable : EnablePort
  Constant : Constant  Value=aij
  Constant1 : Constant  Value=R_in
  Constant12 : Constant  Value=L_in
  Constant13 : Constant  Value=Mpw
  Constant15 : Constant  Value=Tsec
  Constant16 : Constant  Value=a
  Constant5 : Constant  Value=lambda3
  Constant6 : Constant  Value=lambda2
  Constant7 : Constant  Value=lambda1
  Constant8 : Constant  Value=w_nom
  Constant9 : Constant  Value=Pmax
  Model Predictive Control 3 : MATLAB Function  SystemSampleTime=Tsamp
      settings: MinAlgLoopOccurrences=on
  x : Outport
  flag : Outport  Port=2
  wires:
  Constant8/1 -> Model Predictive Control 3/12(w_nom)
  V_s/1 -> Model Predictive Control 3/9(V_s)
  P/1 -> Model Predictive Control 3/11(P)
  omega_s/1 -> Model Predictive Control 3/7(omega_s)
  Constant/1 -> Model Predictive Control 3/17(aij)
  Constant15/1 -> Model Predictive Control 3/5(Tsec)
  omega/1 -> Model Predictive Control 3/6(omega)
  Model Predictive Control 3/2(x_out) -> x/1
  Constant16/1 -> Model Predictive Control 3/2(a)
  Constant13/1 -> Model Predictive Control 3/4(Mpw)
  X/1 -> Model Predictive Control 3/1(X)
  Constant12/1 -> Model Predictive Control 3/3(L_in)
  Constant9/1 -> Model Predictive Control 3/16(Pmax)
  Constant7/1 -> Model Predictive Control 3/13(lambda1)
  Constant5/1 -> Model Predictive Control 3/15(lambda3)
  V/1 -> Model Predictive Control 3/8(V)
  theta/1 -> Model Predictive Control 3/10(theta)
  Constant6/1 -> Model Predictive Control 3/14(lambda2)
  Model Predictive Control 3/1(flag) -> flag/1
  Constant1/1 -> Model Predictive Control 3/18(R_in)

== system Simulation_NoVI/Voltage Source Inverter 1/3to2 3 ==
  "single " : Inport
  "wt " : Inport  Port=2
  Add1 : Sum  Inputs=+++
  Constant2 : Constant  Value=2*pi/3
  Constant3 : Constant  Value=4*pi/3
  Constant4 : Constant  Value=exp(i*2*pi/3)
  Constant5 : Constant  Value=2/3
  Cos : Trigonometry  Operator=cos
  Cos1 : Trigonometry  Operator=cos
  Cos2 : Trigonometry  Operator=cos
  Math Function1 : Math  Operator=square  SignedPower=on
  Mux : Mux  Inputs=3
  Product{3..8} (6 alike) : Product  RndMeth=Zero
  Scope : Scope  NumInputPorts=3
  Sum : Sum  Inputs=|++
  Sum1 : Sum  Inputs=|++
  threePhase : Outport  VectorParamsAs1DForOutWhenUnconnected=off
  wires:
  "single "/1 -> Product5/1, Product4/1, Product3/1
  Cos/1 -> Product3/2
  Constant2/1 -> Sum/2
  Sum/1 -> Cos1/1
  Cos1/1 -> Product4/2
  "wt "/1 -> Sum1/1, Sum/1, Cos/1
  Constant3/1 -> Sum1/2
  Sum1/1 -> Cos2/1
  Cos2/1 -> Product5/2
  Constant4/1 -> Product7/1, Math Function1/1
  Product7/1 -> Add1/2
  Add1/1 -> Product6/1
  Product8/1 -> Add1/3
  Product5/1 -> Scope/3, Mux/3, Product8/2
  Product3/1 -> Scope/1, Mux/1, Add1/1
  Constant5/1 -> Product6/2
  Product4/1 -> Scope/2, Mux/2, Product7/2
  Math Function1/1 -> Product8/1
  Mux/1 -> threePhase/1

== system Simulation_NoVI/Voltage Source Inverter 1/Droop for secondary control2 ==
  P : Inport
  w_nom : Inport  Port=2
  V_nom : Inport  Port=3
  Q : Inport  Port=4
  Gain4 : Gain  Gain=n_q
  Gain5 : Gain  Gain=m_p
  Integrator : Integrator  WrapState=on  WrappedStateUpperValue=2*pi  WrappedStateLowerValue=0
  Sum1 : Sum  Inputs=|+-
  Sum2 : Sum  Inputs=|+-
  Vref : Outport
  wt : Outport  Port=2
  wo : Outport  Port=3
  wires:
  P/1 -> Gain5/1
  w_nom/1 -> Sum2/1
  Gain5/1 -> Sum2/2
  Sum2/1 -> wo/1, Integrator/1  "w"
  Integrator/1 -> wt/1
  V_nom/1 -> Sum1/1  "Vod_s"
  Gain4/1 -> Sum1/2
  Q/1 -> Gain4/1
  Sum1/1 -> Vref/1  "Vod_s"

== system Simulation_NoVI/Voltage Source Inverter 1/Low-pass filter ==
  p_hat : Inport
  q_hat : Inport  Port=2
  Low-Pass Filter (Discrete or Continuous) : eeGeneralControl/Low-Pass Filter (Discrete or Continuous)  K=1  T=lo_co  B=inf  A=-inf  init_option=Inherited from block input  x0=0  Ts=-1
  Low-Pass Filter (Discrete or Continuous)1 : eeGeneralControl/Low-Pass Filter (Discrete or Continuous)  K=1  T=lo_co  B=inf  A=-inf  init_option=Inherited from block input  x0=0  Ts=-1
  P : Outport
  Q : Outport  Port=2
  wires:
  q_hat/1 -> Low-Pass Filter (Discrete or Continuous)1/1
  Low-Pass Filter (Discrete or Continuous)1/1 -> Q/1  "Q"
  Low-Pass Filter (Discrete or Continuous)/1 -> P/1  "P"
  p_hat/1 -> Low-Pass Filter (Discrete or Continuous)/1

== system Simulation_NoVI/Voltage Source Inverter 1/PLL_1p1 ==
  v : Inport
  2pi : Constant  Value=2*pi
  Low-Pass Filter (Discrete or Continuous) : eeGeneralControl/Low-Pass Filter (Discrete or Continuous)  K=1  T=lo_co  B=inf  A=-inf  init_option=Inherited from block input  x0=0  Ts=-1
  PID Controller : slpidlib/PID Controller  Controller=PI  Form=Parallel  TimeDomain=Continuous-time  UseExternalTs=off  SampleTime=-1  IntegratorMethod=Forward Euler  FilterMethod=Forward Euler  ControllerParametersSource=internal  P=100.15925  I=9869  UseKiTs=off  D=0  N=100  UseFilter=on  TunerSelectOption=Transfer Function Based (PID Tuner App)  InitialConditionSource=internal  InitialConditionForIntegrator=0  InitialConditionForFilter=0  DifferentiatorICPrevScaledInput=0  ExternalReset=none  TrackingMode=off  Kt=1  LimitOutput=off  SatLimitsSource=internal  UpperSaturationLimit=inf  LowerSaturationLimit=-inf  LinearizeAsGain=off  AntiWindupMode=none  Kb=1  LimitIntegrator=off  UpperIntegratorSaturationLimit=inf  LowerIntegratorSaturationLimit=-inf  POutMin=[]  POutMax=[]  IOutMin=[]  IOutMax=[]  DOutMin=[]  DOutMax=[]  NOutMin=[]  NOutMax=[]  SumOutMin=[]  SumOutMax=[]  SaturationOutMin=[]  SaturationOutMax=[]  PParamMin=[]  PParamMax=[]  IParamMin=[]  IParamMax=[]  DParamMin=[]  DParamMax=[]  NParamMin=[]  NParamMax=[]  KbParamMin=[]  KbParamMax=[]  KtParamMin=[]  KtParamMax=[]  KbOutMin=[]  KbOutMax=[]  KtOutMin=[]  KtOutMax=[]  IntegratorOutMin=[]  IntegratorOutMax=[]  FilterOutMin=[]  FilterOutMax=[]  SumI1OutMin=[]  SumI1OutMax=[]  SumI2OutMin=[]  SumI2OutMax=[]  SumI3OutMin=[]  SumI3OutMax=[]  SumI4OutMin=[]  SumI4OutMax=[]  SumDOutMin=[]  SumDOutMax=[]  DifferentiatorOutMin=[]  DifferentiatorOutMax=[]  FilterDiffOutCoefMin=[]  FilterDiffOutCoefMax=[]  ReciprocalOutMin=[]  ReciprocalOutMax=[]  SumDenOutMin=[]  SumDenOutMax=[]  SumNumOutMin=[]  SumNumOutMax=[]  DivideOutMin=[]  DivideOutMax=[]  UdiffTsProdOutMin=[]  UdiffTsProdOutMax=[]  NTsProdOutMin=[]  NTsProdOutMax=[]  UintegralTsProdOutMin=[]  UintegralTsProdOutMax=[]  UngainTsProdOutMin=[]  UngainTsProdOutMax=[]  ClampingZeroOutDataTypeStr=Inherit: Inherit via back propagation  ClampingZeroOutMin=[]  ClampingZeroOutMax=[]  FilterDenConstantOutDataTypeStr=Inherit: Inherit via back propagation  FilterDenConstantOutMin=[]  FilterDenConstantOutMax=[]  PCopyOutDataTypeStr=Inherit: Inherit via back propagation  PCopyOutMin=[]  PCopyOutMax=[]  NCopyOutDataTypeStr=Inherit: Inherit via back propagation  NCopyOutMin=[]  NCopyOutMax=[]  IntegratorContinuousStateAttributes=''  IntegratorStateMustResolveToSignalObject=off  IntegratorRTWStateStorageClass=Auto  FilterContinuousStateAttributes=''  FilterStateMustResolveToSignalObject=off  FilterRTWStateStorageClass=Auto  ParallelPVariant=InternalParameters  IdealPVariant=Disabled  IVariant=InternalParameters  DVariant=Disabled  IntegratorVariant=Continuous  SatVariant=Disabled  AWVariant=Passthrough  PCopyVariant=Disabled  TRVariant=Disabled  FdbkBlocksVariant=Forward  IdealPFdbkVariant=Disabled  SatFdbkVariant=Disabled  DerivativeFilterVariant=Disabled  NVariant=Disabled  NCopyVariant=Disabled_SignalSpec  FilterICVariant=Disabled  IntegratorICVariant=InternalICs  ExternalResetVariant=Disabled  TRSumVariant=Passthrough  SumFdbkVariant=Disabled  SumVariant=Sum_PI  TsampFilterVariant=InternalTs  TsampNgainVariant=Passthrough  TsampIntegralVariant=Passthrough  ExternalSaturationOutDataTypeStr=Inherit: Same as second input
  Reset1 : RelationalOperator  OutDataTypeStr=boolean  InputSameDT=off
  Scope : Scope
  Sqrt : Sqrt
  Square : Math  Operator=square
  Square1 : Math  Operator=square
  Sum : Sum  Inputs=|++
  Sum1 : Sum  Inputs=|++
  TienXuly : Subsystem  mask{k=0.5, fc1=50, fc2=10}
      mask prompts: k "he so k"; fc1 "Tan so cat cua bo loc bac 2"; fc2 "Tan so cat cua bo loc thong thap"
  Tinhtheta : Integrator  ExternalReset=rising  UpperSaturationLimit=2*pi
  apha-beta=>dq : Subsystem
  wff : Constant  Value=50*2*pi
  v_dq : Outport
  omega : Outport  Port=2
  wires:
  PID Controller/1 -> Sum1/1
  v/1 -> TienXuly/1(v)
  Tinhtheta/1 -> apha-beta=>dq/1(Theta), Reset1/1
  TienXuly/2(v'q) -> apha-beta=>dq/3(Ubeta)
  apha-beta=>dq/1(vq) -> Square1/1, PID Controller/1
  TienXuly/1(v') -> apha-beta=>dq/2(Uapha)
  2pi/1 -> Reset1/2
  wff/1 -> Sum1/2
  Reset1/1 -> Tinhtheta/2
  apha-beta=>dq/2(vd) -> Square/1
  Square/1 -> Sum/1
  Square1/1 -> Sum/2
  Sum/1 -> Sqrt/1
  Sqrt/1 -> v_dq/1
  Sum1/1 -> Low-Pass Filter (Discrete or Continuous)/1, Tinhtheta/1  "P"
  Low-Pass Filter (Discrete or Continuous)/1 -> Scope/1, omega/1  "P"

== system Simulation_NoVI/Voltage Source Inverter 1/PLL_1p2 ==
  v : Inport
  2pi : Constant  Value=2*pi
  Low-Pass Filter (Discrete or Continuous) : eeGeneralControl/Low-Pass Filter (Discrete or Continuous)  K=1  T=lo_co  B=inf  A=-inf  init_option=Inherited from block input  x0=0  Ts=-1
  PID Controller : slpidlib/PID Controller  Controller=PI  Form=Parallel  TimeDomain=Continuous-time  UseExternalTs=off  SampleTime=-1  IntegratorMethod=Forward Euler  FilterMethod=Forward Euler  ControllerParametersSource=internal  P=100.15925  I=9869  UseKiTs=off  D=0  N=100  UseFilter=on  TunerSelectOption=Transfer Function Based (PID Tuner App)  InitialConditionSource=internal  InitialConditionForIntegrator=0  InitialConditionForFilter=0  DifferentiatorICPrevScaledInput=0  ExternalReset=none  TrackingMode=off  Kt=1  LimitOutput=off  SatLimitsSource=internal  UpperSaturationLimit=inf  LowerSaturationLimit=-inf  LinearizeAsGain=off  AntiWindupMode=none  Kb=1  LimitIntegrator=off  UpperIntegratorSaturationLimit=inf  LowerIntegratorSaturationLimit=-inf  POutMin=[]  POutMax=[]  IOutMin=[]  IOutMax=[]  DOutMin=[]  DOutMax=[]  NOutMin=[]  NOutMax=[]  SumOutMin=[]  SumOutMax=[]  SaturationOutMin=[]  SaturationOutMax=[]  PParamMin=[]  PParamMax=[]  IParamMin=[]  IParamMax=[]  DParamMin=[]  DParamMax=[]  NParamMin=[]  NParamMax=[]  KbParamMin=[]  KbParamMax=[]  KtParamMin=[]  KtParamMax=[]  KbOutMin=[]  KbOutMax=[]  KtOutMin=[]  KtOutMax=[]  IntegratorOutMin=[]  IntegratorOutMax=[]  FilterOutMin=[]  FilterOutMax=[]  SumI1OutMin=[]  SumI1OutMax=[]  SumI2OutMin=[]  SumI2OutMax=[]  SumI3OutMin=[]  SumI3OutMax=[]  SumI4OutMin=[]  SumI4OutMax=[]  SumDOutMin=[]  SumDOutMax=[]  DifferentiatorOutMin=[]  DifferentiatorOutMax=[]  FilterDiffOutCoefMin=[]  FilterDiffOutCoefMax=[]  ReciprocalOutMin=[]  ReciprocalOutMax=[]  SumDenOutMin=[]  SumDenOutMax=[]  SumNumOutMin=[]  SumNumOutMax=[]  DivideOutMin=[]  DivideOutMax=[]  UdiffTsProdOutMin=[]  UdiffTsProdOutMax=[]  NTsProdOutMin=[]  NTsProdOutMax=[]  UintegralTsProdOutMin=[]  UintegralTsProdOutMax=[]  UngainTsProdOutMin=[]  UngainTsProdOutMax=[]  ClampingZeroOutDataTypeStr=Inherit: Inherit via back propagation  ClampingZeroOutMin=[]  ClampingZeroOutMax=[]  FilterDenConstantOutDataTypeStr=Inherit: Inherit via back propagation  FilterDenConstantOutMin=[]  FilterDenConstantOutMax=[]  PCopyOutDataTypeStr=Inherit: Inherit via back propagation  PCopyOutMin=[]  PCopyOutMax=[]  NCopyOutDataTypeStr=Inherit: Inherit via back propagation  NCopyOutMin=[]  NCopyOutMax=[]  IntegratorContinuousStateAttributes=''  IntegratorStateMustResolveToSignalObject=off  IntegratorRTWStateStorageClass=Auto  FilterContinuousStateAttributes=''  FilterStateMustResolveToSignalObject=off  FilterRTWStateStorageClass=Auto  ParallelPVariant=InternalParameters  IdealPVariant=Disabled  IVariant=InternalParameters  DVariant=Disabled  IntegratorVariant=Continuous  SatVariant=Disabled  AWVariant=Passthrough  PCopyVariant=Disabled  TRVariant=Disabled  FdbkBlocksVariant=Forward  IdealPFdbkVariant=Disabled  SatFdbkVariant=Disabled  DerivativeFilterVariant=Disabled  NVariant=Disabled  NCopyVariant=Disabled_SignalSpec  FilterICVariant=Disabled  IntegratorICVariant=InternalICs  ExternalResetVariant=Disabled  TRSumVariant=Passthrough  SumFdbkVariant=Disabled  SumVariant=Sum_PI  TsampFilterVariant=InternalTs  TsampNgainVariant=Passthrough  TsampIntegralVariant=Passthrough  ExternalSaturationOutDataTypeStr=Inherit: Same as second input
  Reset1 : RelationalOperator  OutDataTypeStr=boolean  InputSameDT=off
  Scope : Scope
  Sqrt : Sqrt
  Square : Math  Operator=square
  Square1 : Math  Operator=square
  Sum : Sum  Inputs=|++
  Sum1 : Sum  Inputs=|++
  TienXuly : Subsystem  mask{k=0.5, fc1=50, fc2=10}
      mask prompts: k "he so k"; fc1 "Tan so cat cua bo loc bac 2"; fc2 "Tan so cat cua bo loc thong thap"
  Tinhtheta : Integrator  ExternalReset=rising  UpperSaturationLimit=2*pi
  apha-beta=>dq : Subsystem
  wff : Constant  Value=50*2*pi
  v_dq : Outport
  omega : Outport  Port=2
  wires:
  PID Controller/1 -> Sum1/1
  v/1 -> TienXuly/1(v)
  Tinhtheta/1 -> apha-beta=>dq/1(Theta), Reset1/1
  TienXuly/2(v'q) -> apha-beta=>dq/3(Ubeta)
  apha-beta=>dq/1(vq) -> Square1/1, PID Controller/1
  TienXuly/1(v') -> apha-beta=>dq/2(Uapha)
  2pi/1 -> Reset1/2
  wff/1 -> Sum1/2
  Reset1/1 -> Tinhtheta/2
  apha-beta=>dq/2(vd) -> Square/1
  Square/1 -> Sum/1
  Square1/1 -> Sum/2
  Sum/1 -> Sqrt/1
  Sqrt/1 -> v_dq/1
  Sum1/1 -> Low-Pass Filter (Discrete or Continuous)/1, Tinhtheta/1  "P"
  Low-Pass Filter (Discrete or Continuous)/1 -> Scope/1, omega/1  "P"

== system Simulation_NoVI/Voltage Source Inverter 1/PMW ==
  REF : Inport
  Tri_signal : Inport  Port=2
  Demux : Demux  Outputs=3
  Mux : Mux  Inputs=6
  NOT : Logic  Operator=NOT  AllPortsSameDT=off  OutDataTypeStr=boolean
  NOT1 : Logic  Operator=NOT  AllPortsSameDT=off  OutDataTypeStr=boolean
  NOT2 : Logic  Operator=NOT  AllPortsSameDT=off  OutDataTypeStr=boolean
  Relational Operator : RelationalOperator  OutDataTypeStr=boolean  RndMeth=Simplest  InputSameDT=off
  Relational Operator1 : RelationalOperator  OutDataTypeStr=boolean  RndMeth=Simplest  InputSameDT=off
  Relational Operator2 : RelationalOperator  OutDataTypeStr=boolean  RndMeth=Simplest  InputSameDT=off
  Scope : Scope
  Scope1 : Scope
  Scope2 : Scope  NumInputPorts=2
  Out1 : Outport
  wires:
  Demux/1 -> Relational Operator/1
  Tri_signal/1 -> Relational Operator1/2, Relational Operator/2, Relational Operator2/2
  Demux/2 -> Relational Operator1/1
  Demux/3 -> Relational Operator2/1
  REF/1 -> Scope1/1, Demux/1
  Relational Operator/1 -> Scope2/1, Mux/1, NOT/1
  NOT/1 -> Scope2/2, Mux/2
  Relational Operator1/1 -> NOT1/1, Mux/3
  NOT1/1 -> Mux/4
  Relational Operator2/1 -> Mux/5, NOT2/1
  NOT2/1 -> Mux/6
  Mux/1 -> Scope/1, Out1/1

== system Simulation_NoVI/Voltage Source Inverter 1/PQ calculator ==
  Vod : Inport
  Voq : Inport  Port=2
  Iod : Inport  Port=3
  Ioq : Inport  Port=4
  Product{,1..3} (4 alike) : Product
  Scope : Scope
  Sum10 : Sum  Inputs=|++
  Sum11 : Sum  Inputs=|+-
  p_hat : Outport
  q_hat : Outport  Port=2
  wires:
  Product3/1 -> Sum11/2
  Product1/1 -> Sum10/2
  Voq/1 -> Product3/1, Product1/1
  Iod/1 -> Product/2, Product3/2
  Product2/1 -> Sum11/1
  Ioq/1 -> Product1/2, Product2/2
  Product/1 -> Sum10/1
  Vod/1 -> Scope/1, Product/1, Product2/1
  Sum11/1 -> q_hat/1  "q_hat"
  Sum10/1 -> p_hat/1  "p_hat"
